simulink model "PRUEBA2"  (R2020a)
settings: Solver=VariableStepAuto  StartTime=0.0  StopTime=20  RelTol=1e-3
libraries: fuzblock x5, simulink x4
settings Model: Creator=ANDRES  LastModifiedBy=ANDRES

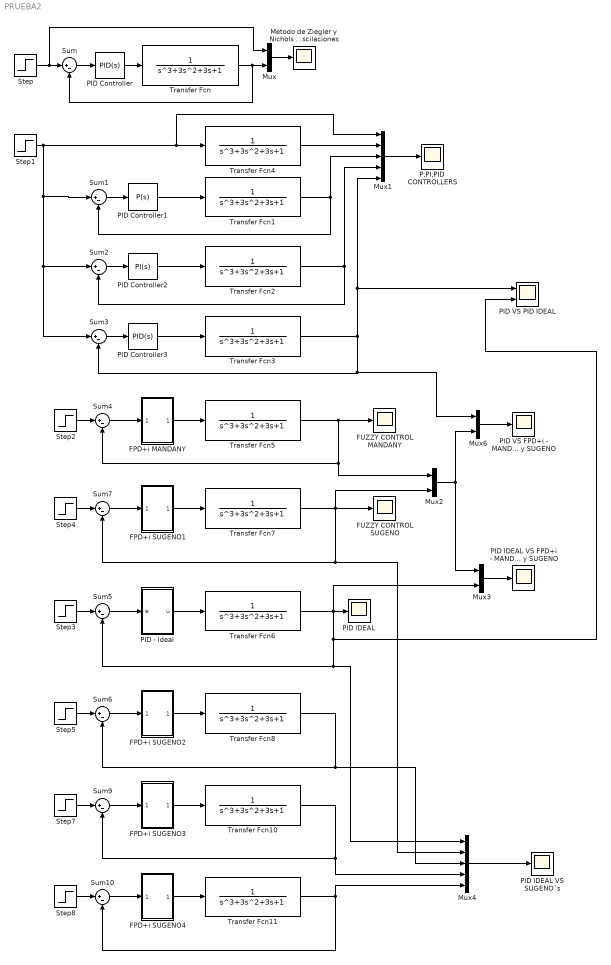
== system PRUEBA2 ==
  FPD+i MANDANY : Subsystem
  FPD+i SUGENO1 : Subsystem
  FPD+i SUGENO2 : Subsystem
  FPD+i SUGENO3 : Subsystem
  FPD+i SUGENO4 : Subsystem
  FUZZY CONTROL MANDANY : Scope
  FUZZY CONTROL SUGENO : Scope
  Metodo de Ziegler y Nichols Oscilaciones : Scope
  Mux{,2..3,6} (4 alike) : Mux  Inputs=2
  Mux1 : Mux  Inputs=5
  Mux4 : Mux  Inputs=5
  P,PI,PID CONTROLLERS : Scope
  PID - Ideal : Subsystem
  PID Controller : simulink/Continuous/PID Controller  Controller=PID  Form=Parallel  TimeDomain=Continuous-time  UseExternalTs=off  SampleTime=-1  IntegratorMethod=Forward Euler  FilterMethod=Forward Euler  ControllerParametersSource=internal  P=8  I=0  D=0  UseFilter=on  N=100  TunerSelectOption=Transfer Function Based (PID Tuner App)  InitialConditionSource=internal  InitialConditionForIntegrator=0  InitialConditionForFilter=0  DifferentiatorICPrevScaledInput=0  ExternalReset=none  TrackingMode=off  Kt=1  LimitOutput=off  UpperSaturationLimit=inf  LowerSaturationLimit=-inf  LinearizeAsGain=on  AntiWindupMode=none  Kb=1  POutMin=[]  POutMax=[]  IOutMin=[]  IOutMax=[]  DOutMin=[]  DOutMax=[]  NOutMin=[]  NOutMax=[]  SumOutMin=[]  SumOutMax=[]  SaturationOutMin=[]  SaturationOutMax=[]  PParamMin=[]  PParamMax=[]  IParamMin=[]  IParamMax=[]  DParamMin=[]  DParamMax=[]  NParamMin=[]  NParamMax=[]  KbParamMin=[]  KbParamMax=[]  KtParamMin=[]  KtParamMax=[]  KbOutMin=[]  KbOutMax=[]  KtOutMin=[]  KtOutMax=[]  IntegratorOutMin=[]  IntegratorOutMax=[]  FilterOutMin=[]  FilterOutMax=[]  SumI1OutMin=[]  SumI1OutMax=[]  SumI2OutMin=[]  SumI2OutMax=[]  SumI3OutMin=[]  SumI3OutMax=[]  SumI4OutMin=[]  SumI4OutMax=[]  SumDOutMin=[]  SumDOutMax=[]  DifferentiatorOutMin=[]  DifferentiatorOutMax=[]  FilterDiffOutCoefMin=[]  FilterDiffOutCoefMax=[]  ReciprocalOutMin=[]  ReciprocalOutMax=[]  SumDenOutMin=[]  SumDenOutMax=[]  SumNumOutMin=[]  SumNumOutMax=[]  DivideOutMin=[]  DivideOutMax=[]  UdiffTsProdOutMin=[]  UdiffTsProdOutMax=[]  NTsProdOutMin=[]  NTsProdOutMax=[]  UintegralTsProdOutMin=[]  UintegralTsProdOutMax=[]  UngainTsProdOutMin=[]  UngainTsProdOutMax=[]  IntegratorContinuousStateAttributes=''  IntegratorStateMustResolveToSignalObject=off  IntegratorRTWStateStorageClass=Auto  FilterContinuousStateAttributes=''  FilterStateMustResolveToSignalObject=off  FilterRTWStateStorageClass=Auto  ParallelPVariant=InternalParameters  IdealPVariant=Disabled  IVariant=InternalParameters  DVariant=InternalParameters  IntegratorVariant=Continuous  SatVariant=Disabled  AWVariant=Passthrough  PCopyVariant=Disabled  TRVariant=Disabled  FdbkBlocksVariant=Forward  IdealPFdbkVariant=Disabled  SatFdbkVariant=Disabled  DerivativeFilterVariant=ContFilter  NVariant=InternalParameters  NCopyVariant=Disabled  FilterICVariant=InternalICsFilter  IntegratorICVariant=InternalICs  ExternalResetVariant=Disabled  TRSumVariant=Passthrough  SumFdbkVariant=Disabled  SumVariant=Sum_PID  TsampFilterVariant=InternalTs  TsampNgainVariant=Passthrough  TsampIntegralVariant=Passthrough
  PID Controller1 : simulink/Continuous/PID Controller  Controller=P  Form=Parallel  TimeDomain=Continuous-time  UseExternalTs=off  SampleTime=-1  IntegratorMethod=Forward Euler  FilterMethod=Forward Euler  ControllerParametersSource=internal  P=4  I=0  D=0  UseFilter=on  N=100  TunerSelectOption=Transfer Function Based (PID Tuner App)  InitialConditionSource=internal  InitialConditionForIntegrator=0  InitialConditionForFilter=0  DifferentiatorICPrevScaledInput=0  ExternalReset=none  TrackingMode=off  Kt=1  LimitOutput=off  UpperSaturationLimit=inf  LowerSaturationLimit=-inf  LinearizeAsGain=on  AntiWindupMode=none  Kb=1  POutMin=[]  POutMax=[]  IOutMin=[]  IOutMax=[]  DOutMin=[]  DOutMax=[]  NOutMin=[]  NOutMax=[]  SumOutMin=[]  SumOutMax=[]  SaturationOutMin=[]  SaturationOutMax=[]  PParamMin=[]  PParamMax=[]  IParamMin=[]  IParamMax=[]  DParamMin=[]  DParamMax=[]  NParamMin=[]  NParamMax=[]  KbParamMin=[]  KbParamMax=[]  KtParamMin=[]  KtParamMax=[]  KbOutMin=[]  KbOutMax=[]  KtOutMin=[]  KtOutMax=[]  IntegratorOutMin=[]  IntegratorOutMax=[]  FilterOutMin=[]  FilterOutMax=[]  SumI1OutMin=[]  SumI1OutMax=[]  SumI2OutMin=[]  SumI2OutMax=[]  SumI3OutMin=[]  SumI3OutMax=[]  SumI4OutMin=[]  SumI4OutMax=[]  SumDOutMin=[]  SumDOutMax=[]  DifferentiatorOutMin=[]  DifferentiatorOutMax=[]  FilterDiffOutCoefMin=[]  FilterDiffOutCoefMax=[]  ReciprocalOutMin=[]  ReciprocalOutMax=[]  SumDenOutMin=[]  SumDenOutMax=[]  SumNumOutMin=[]  SumNumOutMax=[]  DivideOutMin=[]  DivideOutMax=[]  UdiffTsProdOutMin=[]  UdiffTsProdOutMax=[]  NTsProdOutMin=[]  NTsProdOutMax=[]  UintegralTsProdOutMin=[]  UintegralTsProdOutMax=[]  UngainTsProdOutMin=[]  UngainTsProdOutMax=[]  IntegratorContinuousStateAttributes=''  IntegratorStateMustResolveToSignalObject=off  IntegratorRTWStateStorageClass=Auto  FilterContinuousStateAttributes=''  FilterStateMustResolveToSignalObject=off  FilterRTWStateStorageClass=Auto  ParallelPVariant=InternalParameters  IdealPVariant=Disabled  IVariant=Disabled  DVariant=Disabled  IntegratorVariant=Disabled  SatVariant=Disabled  AWVariant=Disabled  PCopyVariant=Disabled  TRVariant=Disabled  FdbkBlocksVariant=Forward  IdealPFdbkVariant=Disabled  SatFdbkVariant=Disabled  DerivativeFilterVariant=Disabled  NVariant=Disabled  NCopyVariant=Disabled_SignalSpec  FilterICVariant=Disabled  IntegratorICVariant=Disabled  ExternalResetVariant=Disabled  TRSumVariant=Passthrough  SumFdbkVariant=Disabled  SumVariant=Passthrough_P  TsampFilterVariant=InternalTs  TsampNgainVariant=Passthrough  TsampIntegralVariant=Disabled_SignalSpec
  PID Controller2 : simulink/Continuous/PID Controller  Controller=PI  Form=Parallel  TimeDomain=Continuous-time  UseExternalTs=off  SampleTime=-1  IntegratorMethod=Forward Euler  FilterMethod=Forward Euler  ControllerParametersSource=internal  P=3.6  I=3.6*(1/3.125)  D=0  UseFilter=on  N=100  TunerSelectOption=Transfer Function Based (PID Tuner App)  InitialConditionSource=internal  InitialConditionForIntegrator=0  InitialConditionForFilter=0  DifferentiatorICPrevScaledInput=0  ExternalReset=none  TrackingMode=off  Kt=1  LimitOutput=off  UpperSaturationLimit=inf  LowerSaturationLimit=-inf  LinearizeAsGain=on  AntiWindupMode=none  Kb=1  POutMin=[]  POutMax=[]  IOutMin=[]  IOutMax=[]  DOutMin=[]  DOutMax=[]  NOutMin=[]  NOutMax=[]  SumOutMin=[]  SumOutMax=[]  SaturationOutMin=[]  SaturationOutMax=[]  PParamMin=[]  PParamMax=[]  IParamMin=[]  IParamMax=[]  DParamMin=[]  DParamMax=[]  NParamMin=[]  NParamMax=[]  KbParamMin=[]  KbParamMax=[]  KtParamMin=[]  KtParamMax=[]  KbOutMin=[]  KbOutMax=[]  KtOutMin=[]  KtOutMax=[]  IntegratorOutMin=[]  IntegratorOutMax=[]  FilterOutMin=[]  FilterOutMax=[]  SumI1OutMin=[]  SumI1OutMax=[]  SumI2OutMin=[]  SumI2OutMax=[]  SumI3OutMin=[]  SumI3OutMax=[]  SumI4OutMin=[]  SumI4OutMax=[]  SumDOutMin=[]  SumDOutMax=[]  DifferentiatorOutMin=[]  DifferentiatorOutMax=[]  FilterDiffOutCoefMin=[]  FilterDiffOutCoefMax=[]  ReciprocalOutMin=[]  ReciprocalOutMax=[]  SumDenOutMin=[]  SumDenOutMax=[]  SumNumOutMin=[]  SumNumOutMax=[]  DivideOutMin=[]  DivideOutMax=[]  UdiffTsProdOutMin=[]  UdiffTsProdOutMax=[]  NTsProdOutMin=[]  NTsProdOutMax=[]  UintegralTsProdOutMin=[]  UintegralTsProdOutMax=[]  UngainTsProdOutMin=[]  UngainTsProdOutMax=[]  IntegratorContinuousStateAttributes=''  IntegratorStateMustResolveToSignalObject=off  IntegratorRTWStateStorageClass=Auto  FilterContinuousStateAttributes=''  FilterStateMustResolveToSignalObject=off  FilterRTWStateStorageClass=Auto  ParallelPVariant=InternalParameters  IdealPVariant=Disabled  IVariant=InternalParameters  DVariant=Disabled  IntegratorVariant=Continuous  SatVariant=Disabled  AWVariant=Passthrough  PCopyVariant=Disabled  TRVariant=Disabled  FdbkBlocksVariant=Forward  IdealPFdbkVariant=Disabled  SatFdbkVariant=Disabled  DerivativeFilterVariant=Disabled  NVariant=Disabled  NCopyVariant=Disabled_SignalSpec  FilterICVariant=Disabled  IntegratorICVariant=InternalICs  ExternalResetVariant=Disabled  TRSumVariant=Passthrough  SumFdbkVariant=Disabled  SumVariant=Sum_PI  TsampFilterVariant=InternalTs  TsampNgainVariant=Passthrough  TsampIntegralVariant=Passthrough
  PID Controller3 : simulink/Continuous/PID Controller  Controller=PID  Form=Parallel  TimeDomain=Continuous-time  UseExternalTs=off  SampleTime=-1  IntegratorMethod=Forward Euler  FilterMethod=Forward Euler  ControllerParametersSource=internal  P=4.8  I=4.8*(1/(15/8))  D=4.8*(15/32)  UseFilter=on  N=100  TunerSelectOption=Transfer Function Based (PID Tuner App)  InitialConditionSource=internal  InitialConditionForIntegrator=0  InitialConditionForFilter=0  DifferentiatorICPrevScaledInput=0  ExternalReset=none  TrackingMode=off  Kt=1  LimitOutput=off  UpperSaturationLimit=inf  LowerSaturationLimit=-inf  LinearizeAsGain=on  AntiWindupMode=none  Kb=1  POutMin=[]  POutMax=[]  IOutMin=[]  IOutMax=[]  DOutMin=[]  DOutMax=[]  NOutMin=[]  NOutMax=[]  SumOutMin=[]  SumOutMax=[]  SaturationOutMin=[]  SaturationOutMax=[]  PParamMin=[]  PParamMax=[]  IParamMin=[]  IParamMax=[]  DParamMin=[]  DParamMax=[]  NParamMin=[]  NParamMax=[]  KbParamMin=[]  KbParamMax=[]  KtParamMin=[]  KtParamMax=[]  KbOutMin=[]  KbOutMax=[]  KtOutMin=[]  KtOutMax=[]  IntegratorOutMin=[]  IntegratorOutMax=[]  FilterOutMin=[]  FilterOutMax=[]  SumI1OutMin=[]  SumI1OutMax=[]  SumI2OutMin=[]  SumI2OutMax=[]  SumI3OutMin=[]  SumI3OutMax=[]  SumI4OutMin=[]  SumI4OutMax=[]  SumDOutMin=[]  SumDOutMax=[]  DifferentiatorOutMin=[]  DifferentiatorOutMax=[]  FilterDiffOutCoefMin=[]  FilterDiffOutCoefMax=[]  ReciprocalOutMin=[]  ReciprocalOutMax=[]  SumDenOutMin=[]  SumDenOutMax=[]  SumNumOutMin=[]  SumNumOutMax=[]  DivideOutMin=[]  DivideOutMax=[]  UdiffTsProdOutMin=[]  UdiffTsProdOutMax=[]  NTsProdOutMin=[]  NTsProdOutMax=[]  UintegralTsProdOutMin=[]  UintegralTsProdOutMax=[]  UngainTsProdOutMin=[]  UngainTsProdOutMax=[]  IntegratorContinuousStateAttributes=''  IntegratorStateMustResolveToSignalObject=off  IntegratorRTWStateStorageClass=Auto  FilterContinuousStateAttributes=''  FilterStateMustResolveToSignalObject=off  FilterRTWStateStorageClass=Auto  ParallelPVariant=InternalParameters  IdealPVariant=Disabled  IVariant=InternalParameters  DVariant=InternalParameters  IntegratorVariant=Continuous  SatVariant=Disabled  AWVariant=Passthrough  PCopyVariant=Disabled  TRVariant=Disabled  FdbkBlocksVariant=Forward  IdealPFdbkVariant=Disabled  SatFdbkVariant=Disabled  DerivativeFilterVariant=ContFilter  NVariant=InternalParameters  NCopyVariant=Disabled  FilterICVariant=InternalICsFilter  IntegratorICVariant=InternalICs  ExternalResetVariant=Disabled  TRSumVariant=Passthrough  SumFdbkVariant=Disabled  SumVariant=Sum_PID  TsampFilterVariant=InternalTs  TsampNgainVariant=Passthrough  TsampIntegralVariant=Passthrough
  PID IDEAL : Scope
  PID IDEAL VS FPD+i - MANDANY y SUGENO : Scope
  PID IDEAL VS SUGENO´s : Scope
  PID VS FPD+i - MANDANY y SUGENO : Scope
  PID VS PID IDEAL : Scope  NumInputPorts=2
  Step{,1..5,7..8} (8 alike) : Step  SampleTime=0
  Sum{,1..7,9..10} (10 alike) : Sum  Inputs=|+-
  Transfer Fcn{,1..8,10..11} (11 alike) : TransferFcn  Denominator=[1 3 3 1]
  wires:
  PID Controller/1 -> Transfer Fcn/1
  Transfer Fcn/1 -> Mux/2, Sum/2
  Sum/1 -> PID Controller/1
  Mux/1 -> Metodo de Ziegler y Nichols Oscilaciones/1
  Step/1 -> Mux/1, Sum/1
  Sum1/1 -> PID Controller1/1
  Transfer Fcn1/1 -> Mux1/3, Sum1/2
  PID Controller1/1 -> Transfer Fcn1/1
  Sum2/1 -> PID Controller2/1
  Transfer Fcn2/1 -> Mux1/4, Sum2/2
  PID Controller2/1 -> Transfer Fcn2/1
  Sum3/1 -> PID Controller3/1
  PID Controller3/1 -> Transfer Fcn3/1
  Step1/1 -> Sum3/1, Sum2/1, Sum1/1, Mux1/1, Transfer Fcn4/1
  FPD+i MANDANY/1(out) -> Transfer Fcn5/1
  Sum4/1 -> FPD+i MANDANY/1(error)
  Step2/1 -> Sum4/1
  Step3/1 -> Sum5/1
  Mux3/1 -> PID IDEAL VS FPD+i - MANDANY y SUGENO/1
  Transfer Fcn3/1 -> PID VS PID IDEAL/1, Mux1/5, Mux6/1, Sum3/2
  Sum7/1 -> FPD+i SUGENO1/1(error)
  FPD+i SUGENO1/1(out) -> Transfer Fcn7/1
  Step4/1 -> Sum7/1
  Transfer Fcn7/1 -> Mux2/2, FUZZY CONTROL SUGENO/1, Sum7/2, Mux4/2
  Mux1/1 -> P,PI,PID CONTROLLERS/1
  Transfer Fcn4/1 -> Mux1/2
  Sum5/1 -> PID - Ideal/1(e)
  PID - Ideal/1(u) -> Transfer Fcn6/1
  Transfer Fcn5/1 -> Mux2/1, Sum4/2, FUZZY CONTROL MANDANY/1
  Mux2/1 -> Mux3/1, Mux6/2
  Mux6/1 -> PID VS FPD+i - MANDANY y SUGENO/1
  FPD+i SUGENO2/1(out) -> Transfer Fcn8/1
  Sum6/1 -> FPD+i SUGENO2/1(error)
  Transfer Fcn8/1 -> Mux4/3, Sum6/2
  Step5/1 -> Sum6/1
  Transfer Fcn10/1 -> Mux4/4, Sum9/2
  Step7/1 -> Sum9/1
  FPD+i SUGENO3/1(out) -> Transfer Fcn10/1
  Sum9/1 -> FPD+i SUGENO3/1(error)
  Transfer Fcn11/1 -> Sum10/2, Mux4/5
  Step8/1 -> Sum10/1
  FPD+i SUGENO4/1(out) -> Transfer Fcn11/1
  Sum10/1 -> FPD+i SUGENO4/1(error)
  Mux4/1 -> PID IDEAL VS SUGENO´s/1
  Transfer Fcn6/1 -> PID IDEAL/1, PID VS PID IDEAL/2, Mux4/1, Sum5/2, Mux3/2

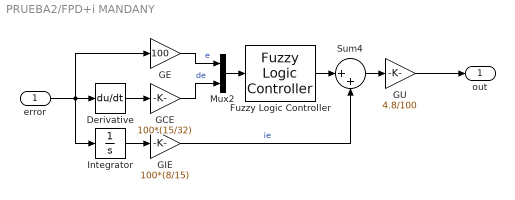
== system PRUEBA2/FPD+i MANDANY ==
  error : Inport
  Derivative : Derivative
  Fuzzy Logic Controller : fuzblock/Fuzzy Logic  Controller  FIS=Fuzzy1  OutputSampleNumber=101  DataType=double  FuzzifiedInputs=off  RuleFiringStrengths=off  RuleOutputs=off  AggregatedOutputs=off  SimulateUsing=Interpreted execution  OutOfRangeInputValueMessage=warning  NoRuleFiredMessage=warning  EmptyOutputFuzzySetMessage=warning
  GCE : Gain  Gain=100*(15/32)
  GE : Gain  Gain=100
  GIE : Gain  Gain=100*(8/15)
  GU : Gain  Gain=4.8/100
  Integrator : Integrator
  Mux2 : Mux  Inputs=2
  Sum4 : Sum  Inputs=|++
  out : Outport  VectorParamsAs1DForOutWhenUnconnected=off
  wires:
  Sum4/1 -> GU/1
  Derivative/1 -> GCE/1
  error/1 -> Integrator/1, GE/1, Derivative/1
  Integrator/1 -> GIE/1
  GCE/1 -> Mux2/2  "de"
  GE/1 -> Mux2/1  "e"
  Mux2/1 -> Fuzzy Logic Controller/1
  GU/1 -> out/1
  Fuzzy Logic Controller/1 -> Sum4/1
  GIE/1 -> Sum4/2  "ie"

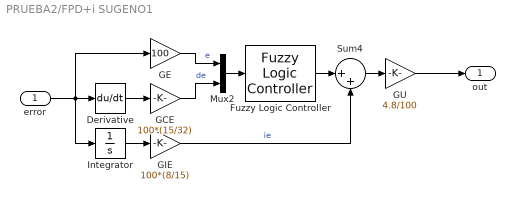
== system PRUEBA2/FPD+i SUGENO1 ==
  error : Inport
  Derivative : Derivative
  Fuzzy Logic Controller : fuzblock/Fuzzy Logic  Controller  FIS=Fuzzy2  OutputSampleNumber=101  DataType=double  FuzzifiedInputs=off  RuleFiringStrengths=off  RuleOutputs=off  AggregatedOutputs=off  SimulateUsing=Interpreted execution  OutOfRangeInputValueMessage=warning  NoRuleFiredMessage=warning  EmptyOutputFuzzySetMessage=warning
  GCE : Gain  Gain=100*(15/32)
  GE : Gain  Gain=100
  GIE : Gain  Gain=100*(8/15)
  GU : Gain  Gain=4.8/100
  Integrator : Integrator
  Mux2 : Mux  Inputs=2
  Sum4 : Sum  Inputs=|++
  out : Outport  VectorParamsAs1DForOutWhenUnconnected=off
  wires:
  Sum4/1 -> GU/1
  Derivative/1 -> GCE/1
  error/1 -> Integrator/1, GE/1, Derivative/1
  Integrator/1 -> GIE/1
  GCE/1 -> Mux2/2  "de"
  GE/1 -> Mux2/1  "e"
  Mux2/1 -> Fuzzy Logic Controller/1
  GU/1 -> out/1
  Fuzzy Logic Controller/1 -> Sum4/1
  GIE/1 -> Sum4/2  "ie"

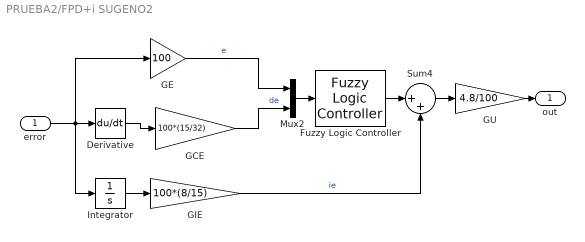
== system PRUEBA2/FPD+i SUGENO2 ==
  error : Inport
  Derivative : Derivative
  Fuzzy Logic Controller : fuzblock/Fuzzy Logic  Controller  FIS=Fuzzy3  OutputSampleNumber=101  DataType=double  FuzzifiedInputs=off  RuleFiringStrengths=off  RuleOutputs=off  AggregatedOutputs=off  SimulateUsing=Interpreted execution  OutOfRangeInputValueMessage=warning  NoRuleFiredMessage=warning  EmptyOutputFuzzySetMessage=warning
  GCE : Gain  Gain=100*(15/32)
  GE : Gain  Gain=100
  GIE : Gain  Gain=100*(8/15)
  GU : Gain  Gain=4.8/100
  Integrator : Integrator
  Mux2 : Mux  Inputs=2
  Sum4 : Sum  Inputs=|++
  out : Outport  VectorParamsAs1DForOutWhenUnconnected=off
  wires:
  Sum4/1 -> GU/1
  Derivative/1 -> GCE/1
  error/1 -> Integrator/1, GE/1, Derivative/1
  Integrator/1 -> GIE/1
  GCE/1 -> Mux2/2  "de"
  GE/1 -> Mux2/1  "e"
  Mux2/1 -> Fuzzy Logic Controller/1
  GU/1 -> out/1
  Fuzzy Logic Controller/1 -> Sum4/1
  GIE/1 -> Sum4/2  "ie"

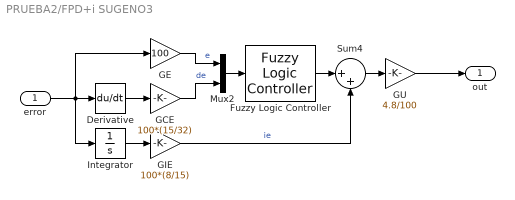
== system PRUEBA2/FPD+i SUGENO3 ==
  error : Inport
  Derivative : Derivative
  Fuzzy Logic Controller : fuzblock/Fuzzy Logic  Controller  FIS=Fuzzy4  OutputSampleNumber=101  DataType=double  FuzzifiedInputs=off  RuleFiringStrengths=off  RuleOutputs=off  AggregatedOutputs=off  SimulateUsing=Interpreted execution  OutOfRangeInputValueMessage=warning  NoRuleFiredMessage=warning  EmptyOutputFuzzySetMessage=warning
  GCE : Gain  Gain=100*(15/32)
  GE : Gain  Gain=100
  GIE : Gain  Gain=100*(8/15)
  GU : Gain  Gain=4.8/100
  Integrator : Integrator
  Mux2 : Mux  Inputs=2
  Sum4 : Sum  Inputs=|++
  out : Outport  VectorParamsAs1DForOutWhenUnconnected=off
  wires:
  Sum4/1 -> GU/1
  Derivative/1 -> GCE/1
  error/1 -> Integrator/1, GE/1, Derivative/1
  Integrator/1 -> GIE/1
  GCE/1 -> Mux2/2  "de"
  GE/1 -> Mux2/1  "e"
  Mux2/1 -> Fuzzy Logic Controller/1
  GU/1 -> out/1
  Fuzzy Logic Controller/1 -> Sum4/1
  GIE/1 -> Sum4/2  "ie"

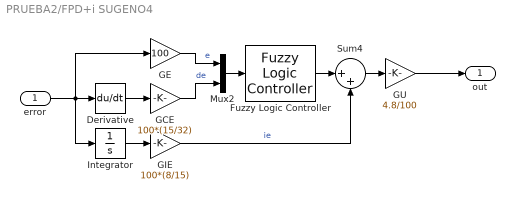
== system PRUEBA2/FPD+i SUGENO4 ==
  error : Inport
  Derivative : Derivative
  Fuzzy Logic Controller : fuzblock/Fuzzy Logic  Controller  FIS=Fuzzy5  OutputSampleNumber=101  DataType=double  FuzzifiedInputs=off  RuleFiringStrengths=off  RuleOutputs=off  AggregatedOutputs=off  SimulateUsing=Interpreted execution  OutOfRangeInputValueMessage=warning  NoRuleFiredMessage=warning  EmptyOutputFuzzySetMessage=warning
  GCE : Gain  Gain=100*(15/32)
  GE : Gain  Gain=100
  GIE : Gain  Gain=100*(8/15)
  GU : Gain  Gain=4.8/100
  Integrator : Integrator
  Mux2 : Mux  Inputs=2
  Sum4 : Sum  Inputs=|++
  out : Outport  VectorParamsAs1DForOutWhenUnconnected=off
  wires:
  Sum4/1 -> GU/1
  Derivative/1 -> GCE/1
  error/1 -> Integrator/1, GE/1, Derivative/1
  Integrator/1 -> GIE/1
  GCE/1 -> Mux2/2  "de"
  GE/1 -> Mux2/1  "e"
  Mux2/1 -> Fuzzy Logic Controller/1
  GU/1 -> out/1
  Fuzzy Logic Controller/1 -> Sum4/1
  GIE/1 -> Sum4/2  "ie"

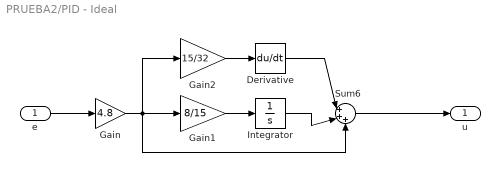
== system PRUEBA2/PID - Ideal ==
  e : Inport
  Derivative : Derivative
  Gain : Gain  Gain=4.8
  Gain1 : Gain  Gain=8/15
  Gain2 : Gain  Gain=15/32
  Integrator : Integrator
  Sum6 : Sum  Inputs=|+++
  u : Outport
  wires:
  Gain1/1 -> Integrator/1
  Derivative/1 -> Sum6/1
  Gain2/1 -> Derivative/1
  Integrator/1 -> Sum6/2
  Gain/1 -> Gain2/1, Gain1/1, Sum6/3
  Sum6/1 -> u/1
  e/1 -> Gain/1
